simulink model "NonlinearNoObserverBlock"  (R2019b)
settings: Solver=VariableStepAuto  StartTime=0.0  StopTime=30  RelTol=1e-3
settings Model: Creator=marko  LastModifiedBy=marko

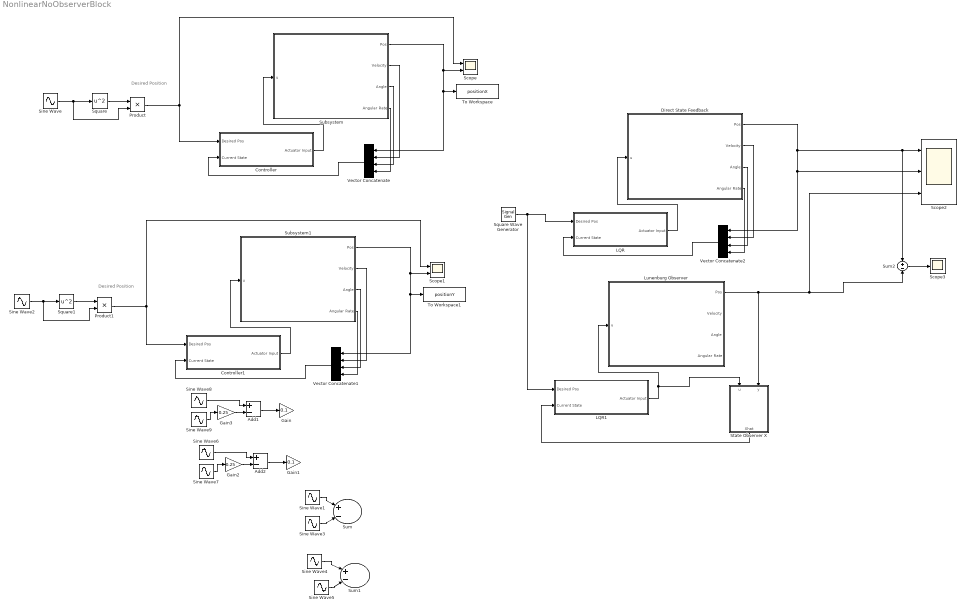
== system NonlinearNoObserverBlock ==
  note: Desired Position
  note: Desired Position
  Add1 : Sum  Inputs=+-
  Add2 : Sum  Inputs=+-
  Controller : Subsystem
  Controller1 : Subsystem
  Direct State Feedback : Subsystem
  Gain : Gain  Gain=0.1
  Gain1 : Gain  Gain=0.1
  Gain2 : Gain  Gain=0.25
  Gain3 : Gain  Gain=0.25
  LQR : Subsystem
  LQR1 : Subsystem
  Lunenburg Observer : Subsystem
  Product : Product
  Product1 : Product
  Scope : Scope  NumInputPorts=2
  Scope1 : Scope  NumInputPorts=2
  Scope2 : Scope  NumInputPorts=3
  Scope3 : Scope
  Sine Wave : Sin  SampleTime=0
  Sine Wave1 : Sin  Amplitude=2  SampleTime=0
  Sine Wave2 : Sin  Phase=pi/2  SampleTime=0
  Sine Wave3 : Sin  Frequency=2  SampleTime=0
  Sine Wave4 : Sin  Amplitude=2  Phase=pi/2  SampleTime=0
  Sine Wave5 : Sin  Frequency=2  Phase=pi/2  SampleTime=0
  Sine Wave6 : Sin  Amplitude=1.25  Phase=pi/2  SampleTime=0
  Sine Wave7 : Sin  Frequency=5  Phase=pi/2  SampleTime=0
  Sine Wave8 : Sin  Amplitude=1.25  Phase=pi/2  SampleTime=0
  Sine Wave9 : Sin  Frequency=5  Phase=pi/2  SampleTime=0
  Square : Math  Operator=square  SignedPower=off  SaturateOnIntegerOverflow=on
  Square Wave Generator : SignalGenerator  WaveForm=square  Amplitude=0.1  Frequency=0.5  Units=rad/sec
  Square1 : Math  Operator=square  SignedPower=off  SaturateOnIntegerOverflow=on
  State Observer X : Subsystem
  Subsystem : Subsystem
  Subsystem1 : Subsystem
  Sum : Sum  Inputs=|+-|
  Sum1 : Sum  Inputs=|+-|
  Sum2 : Sum  Inputs=+-
  To Workspace : ToWorkspace  VariableName=positionX  SampleTime=-1
  To Workspace1 : ToWorkspace  VariableName=positionY  SampleTime=-1
  Vector Concatenate : Concatenate  NumInputs=4
  Vector Concatenate1 : Concatenate  NumInputs=4
  Vector Concatenate2 : Concatenate  NumInputs=4
  wires:
  Subsystem/1(Pos) -> Scope/2, Vector Concatenate/1, To Workspace/1
  Controller/1(Actuator Input) -> Subsystem/1(u)
  Square1/1 -> Product1/1
  Product/1 -> Scope/1, Controller/1(Desired Pos)
  Sine Wave2/1 -> Product1/2, Square1/1
  Sine Wave4/1 -> Sum1/1
  Sine Wave3/1 -> Sum/2
  Sine Wave1/1 -> Sum/1
  Square/1 -> Product/1
  Sine Wave5/1 -> Sum1/2
  Sine Wave/1 -> Product/2, Square/1
  Vector Concatenate/1 -> Controller/2(Current State)
  Subsystem/2(Velocity) -> Vector Concatenate/2
  Subsystem/3(Angle) -> Vector Concatenate/3
  Subsystem/4(Angular Rate) -> Vector Concatenate/4
  Product1/1 -> Controller1/1(Desired Pos), Scope1/1
  Controller1/1(Actuator Input) -> Subsystem1/1(u)
  Vector Concatenate1/1 -> Controller1/2(Current State)
  Subsystem1/4(Angular Rate) -> Vector Concatenate1/4
  Subsystem1/1(Pos) -> Scope1/2, To Workspace1/1, Vector Concatenate1/1
  Subsystem1/3(Angle) -> Vector Concatenate1/3
  Subsystem1/2(Velocity) -> Vector Concatenate1/2
  Sine Wave7/1 -> Gain2/1
  Add2/1 -> Gain1/1
  Gain2/1 -> Add2/2
  Sine Wave6/1 -> Add2/1
  Gain3/1 -> Add1/2
  Sine Wave8/1 -> Add1/1
  Add1/1 -> Gain/1
  Sine Wave9/1 -> Gain3/1
  Direct State Feedback/3(Angle) -> Vector Concatenate2/3
  Direct State Feedback/2(Velocity) -> Vector Concatenate2/2
  LQR/1(Actuator Input) -> Direct State Feedback/1(u)
  Vector Concatenate2/1 -> LQR/2(Current State)
  Direct State Feedback/4(Angular Rate) -> Vector Concatenate2/4
  Direct State Feedback/1(Pos) -> Vector Concatenate2/1, Scope2/2, Sum2/1, Scope2/1
  LQR1/1(Actuator Input) -> State Observer X/1(u), Lunenburg Observer/1(u)
  State Observer X/1(Xhat) -> LQR1/2(Current State)
  Lunenburg Observer/1(Pos) -> State Observer X/2(y), Scope2/3, Sum2/2
  Sum2/1 -> Scope3/1
  Square Wave Generator/1 -> LQR1/1(Desired Pos), LQR/1(Desired Pos)

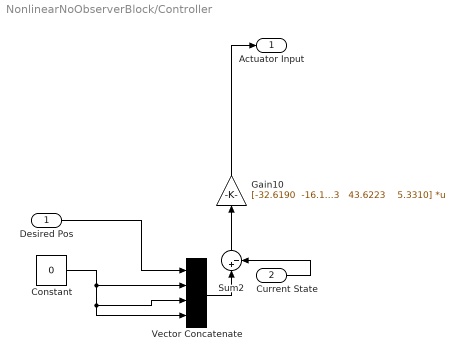
== system NonlinearNoObserverBlock/Controller ==
  Desired Pos : Inport
  Current State : Inport  Port=2
  Constant : Constant  Value=0
  Gain10 : Gain  Gain="[-32.6190  -16.1083   43.6223    5.3310]"  Multiplication=Matrix(K*u)
  Sum2 : Sum  Inputs=|+-
  Vector Concatenate : Concatenate  NumInputs=4
  Actuator Input : Outport
  wires:
  Desired Pos/1 -> Vector Concatenate/1
  Gain10/1 -> Actuator Input/1
  Constant/1 -> Vector Concatenate/2, Vector Concatenate/4, Vector Concatenate/3
  Current State/1 -> Sum2/2
  Sum2/1 -> Gain10/1
  Vector Concatenate/1 -> Sum2/1

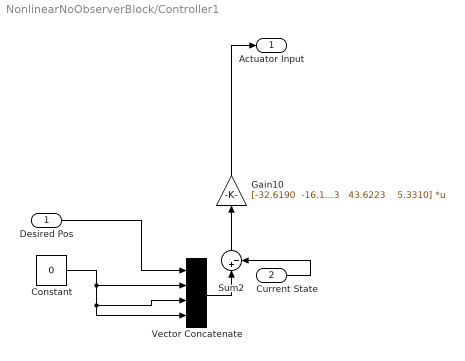
== system NonlinearNoObserverBlock/Controller1 ==
  Desired Pos : Inport
  Current State : Inport  Port=2
  Constant : Constant  Value=0
  Gain10 : Gain  Gain="[-32.6190  -16.1083   43.6223    5.3310]"  Multiplication=Matrix(K*u)
  Sum2 : Sum  Inputs=|+-
  Vector Concatenate : Concatenate  NumInputs=4
  Actuator Input : Outport
  wires:
  Desired Pos/1 -> Vector Concatenate/1
  Gain10/1 -> Actuator Input/1
  Constant/1 -> Vector Concatenate/2, Vector Concatenate/4, Vector Concatenate/3
  Current State/1 -> Sum2/2
  Sum2/1 -> Gain10/1
  Vector Concatenate/1 -> Sum2/1

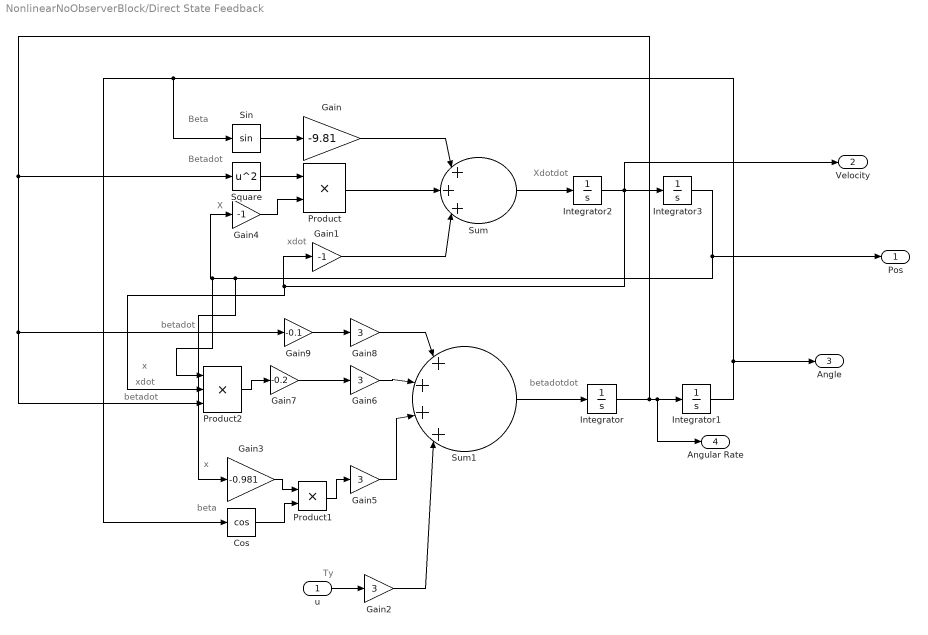
== system NonlinearNoObserverBlock/Direct State Feedback ==
  note: betadotdot
  note: betadot
  note: betadot
  note: xdot
  note: x
  note: beta
  note: x
  note: Ty
  note: xdot
  note: X
  note: Betadot
  note: Beta
  note: Xdotdot
  u : Inport
  Cos : Trigonometry  Operator=cos
  Gain : Gain  Gain=-9.81
  Gain1 : Gain  Gain=-1
  Gain{2,5..6,8} (4 alike) : Gain  Gain=3
  Gain3 : Gain  Gain=-0.981
  Gain4 : Gain  Gain=-1
  Gain7 : Gain  Gain=-0.2
  Gain9 : Gain  Gain=-0.1
  Integrator{,1..3} (4 alike) : Integrator
  Product : Product
  Product1 : Product
  Product2 : Product  Inputs=3
  Sin : Trigonometry
  Square : Math  Operator=square  SignedPower=off  SaturateOnIntegerOverflow=on
  Sum : Sum  Inputs=|+++|
  Sum1 : Sum  Inputs=|++++|
  Pos : Outport
  Velocity : Outport  Port=2
  Angle : Outport  Port=3
  Angular Rate : Outport  Port=4
  wires:
  Gain2/1 -> Sum1/4
  Gain8/1 -> Sum1/1
  Sum1/1 -> Integrator/1
  Integrator3/1 -> Pos/1, Gain3/1, Product2/1, Gain4/1
  Product1/1 -> Gain5/1
  Gain1/1 -> Sum/3
  Product/1 -> Sum/2
  Gain4/1 -> Product/2
  Sum/1 -> Integrator2/1
  Square/1 -> Product/1
  Gain3/1 -> Product1/1
  Gain6/1 -> Sum1/2
  Gain9/1 -> Gain8/1
  Gain/1 -> Sum/1
  Cos/1 -> Product1/2
  Integrator/1 -> Gain9/1, Product2/3, Square/1, Angular Rate/1, Integrator1/1
  Integrator1/1 -> Angle/1, Cos/1, Sin/1
  Gain5/1 -> Sum1/3
  Gain7/1 -> Gain6/1
  Sin/1 -> Gain/1
  Integrator2/1 -> Velocity/1, Product2/2, Gain1/1, Integrator3/1
  Product2/1 -> Gain7/1
  u/1 -> Gain2/1

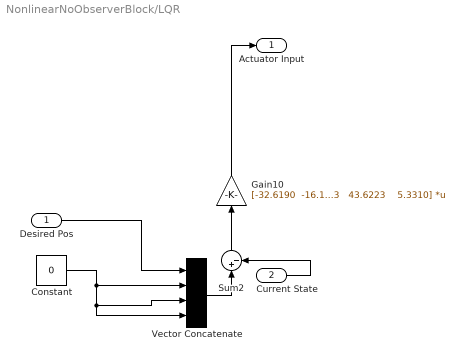
== system NonlinearNoObserverBlock/LQR ==
  Desired Pos : Inport
  Current State : Inport  Port=2
  Constant : Constant  Value=0
  Gain10 : Gain  Gain="[-32.6190  -16.1083   43.6223    5.3310]"  Multiplication=Matrix(K*u)
  Sum2 : Sum  Inputs=|+-
  Vector Concatenate : Concatenate  NumInputs=4
  Actuator Input : Outport
  wires:
  Desired Pos/1 -> Vector Concatenate/1
  Gain10/1 -> Actuator Input/1
  Constant/1 -> Vector Concatenate/2, Vector Concatenate/4, Vector Concatenate/3
  Current State/1 -> Sum2/2
  Sum2/1 -> Gain10/1
  Vector Concatenate/1 -> Sum2/1

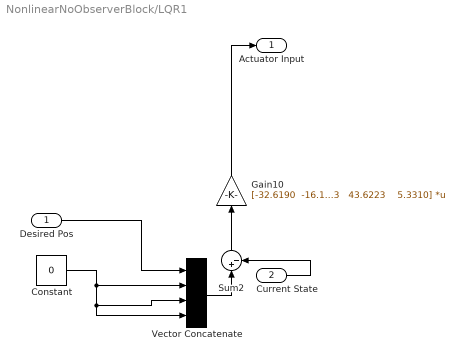
== system NonlinearNoObserverBlock/LQR1 ==
  Desired Pos : Inport
  Current State : Inport  Port=2
  Constant : Constant  Value=0
  Gain10 : Gain  Gain="[-32.6190  -16.1083   43.6223    5.3310]"  Multiplication=Matrix(K*u)
  Sum2 : Sum  Inputs=|+-
  Vector Concatenate : Concatenate  NumInputs=4
  Actuator Input : Outport
  wires:
  Desired Pos/1 -> Vector Concatenate/1
  Gain10/1 -> Actuator Input/1
  Constant/1 -> Vector Concatenate/2, Vector Concatenate/4, Vector Concatenate/3
  Current State/1 -> Sum2/2
  Sum2/1 -> Gain10/1
  Vector Concatenate/1 -> Sum2/1

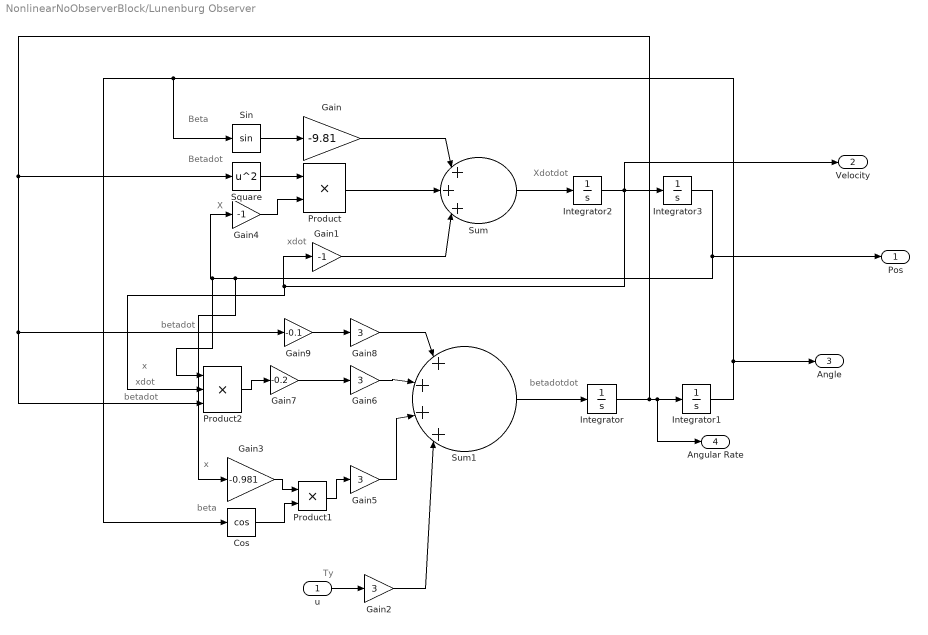
== system NonlinearNoObserverBlock/Lunenburg Observer ==
  note: betadotdot
  note: betadot
  note: betadot
  note: xdot
  note: x
  note: beta
  note: x
  note: Ty
  note: xdot
  note: X
  note: Betadot
  note: Beta
  note: Xdotdot
  u : Inport
  Cos : Trigonometry  Operator=cos
  Gain : Gain  Gain=-9.81
  Gain1 : Gain  Gain=-1
  Gain{2,5..6,8} (4 alike) : Gain  Gain=3
  Gain3 : Gain  Gain=-0.981
  Gain4 : Gain  Gain=-1
  Gain7 : Gain  Gain=-0.2
  Gain9 : Gain  Gain=-0.1
  Integrator{,1..3} (4 alike) : Integrator
  Product : Product
  Product1 : Product
  Product2 : Product  Inputs=3
  Sin : Trigonometry
  Square : Math  Operator=square  SignedPower=off  SaturateOnIntegerOverflow=on
  Sum : Sum  Inputs=|+++|
  Sum1 : Sum  Inputs=|++++|
  Pos : Outport
  Velocity : Outport  Port=2
  Angle : Outport  Port=3
  Angular Rate : Outport  Port=4
  wires:
  Gain2/1 -> Sum1/4
  Gain8/1 -> Sum1/1
  Sum1/1 -> Integrator/1
  Integrator3/1 -> Pos/1, Gain3/1, Product2/1, Gain4/1
  Product1/1 -> Gain5/1
  Gain1/1 -> Sum/3
  Product/1 -> Sum/2
  Gain4/1 -> Product/2
  Sum/1 -> Integrator2/1
  Square/1 -> Product/1
  Gain3/1 -> Product1/1
  Gain6/1 -> Sum1/2
  Gain9/1 -> Gain8/1
  Gain/1 -> Sum/1
  Cos/1 -> Product1/2
  Integrator/1 -> Gain9/1, Product2/3, Square/1, Angular Rate/1, Integrator1/1
  Integrator1/1 -> Angle/1, Cos/1, Sin/1
  Gain5/1 -> Sum1/3
  Gain7/1 -> Gain6/1
  Sin/1 -> Gain/1
  Integrator2/1 -> Velocity/1, Product2/2, Gain1/1, Integrator3/1
  Product2/1 -> Gain7/1
  u/1 -> Gain2/1

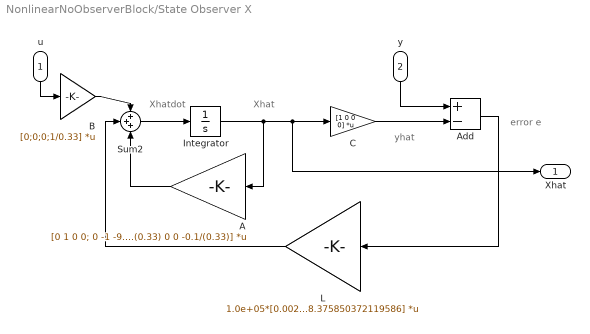
== system NonlinearNoObserverBlock/State Observer X ==
  note: Xhat
  note: error e
  note: yhat
  note: Xhatdot
  u : Inport
  y : Inport  Port=2
  A : Gain  Gain=[0 1 0 0; 0 -1 -9.8 0; 0 0 0 1; -0.98/(0.33) 0 0 -0.1/(0.33)]  Multiplication=Matrix(K*u)
  Add : Sum  Inputs=+-
  B : Gain  Gain=[0;0;0;1/0.33]  Multiplication=Matrix(K*u)
  C : Gain  Gain=[1 0 0 0]  Multiplication=Matrix(K*u)
  Integrator : Integrator  InitialCondition=[0;0;0;0]
  L : Gain  Gain=1.0e+05*[0.002186969696867;0.176147281894242; -0.645506052740811;-8.375850372119586]  Multiplication=Matrix(K*u)
  Sum2 : Sum  Inputs=+++
  Xhat : Outport
  wires:
  B/1 -> Sum2/1
  L/1 -> Sum2/2
  Integrator/1 -> A/1, C/1, Xhat/1
  Sum2/1 -> Integrator/1
  A/1 -> Sum2/3
  u/1 -> B/1
  C/1 -> Add/2
  y/1 -> Add/1
  Add/1 -> L/1

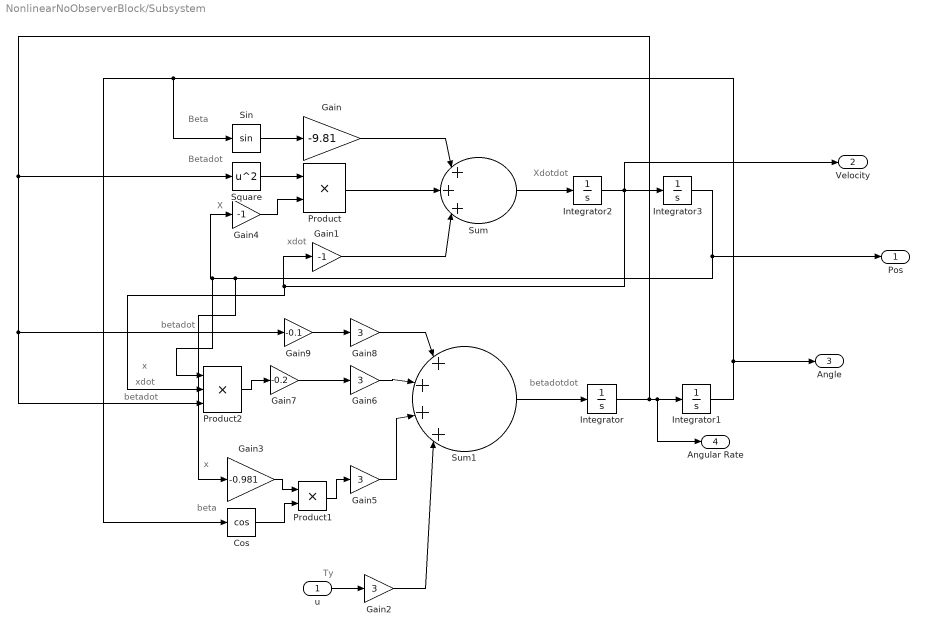
== system NonlinearNoObserverBlock/Subsystem ==
  note: betadotdot
  note: betadot
  note: betadot
  note: xdot
  note: x
  note: beta
  note: x
  note: Ty
  note: xdot
  note: X
  note: Betadot
  note: Beta
  note: Xdotdot
  u : Inport
  Cos : Trigonometry  Operator=cos
  Gain : Gain  Gain=-9.81
  Gain1 : Gain  Gain=-1
  Gain{2,5..6,8} (4 alike) : Gain  Gain=3
  Gain3 : Gain  Gain=-0.981
  Gain4 : Gain  Gain=-1
  Gain7 : Gain  Gain=-0.2
  Gain9 : Gain  Gain=-0.1
  Integrator{,1..3} (4 alike) : Integrator
  Product : Product
  Product1 : Product
  Product2 : Product  Inputs=3
  Sin : Trigonometry
  Square : Math  Operator=square  SignedPower=off  SaturateOnIntegerOverflow=on
  Sum : Sum  Inputs=|+++|
  Sum1 : Sum  Inputs=|++++|
  Pos : Outport
  Velocity : Outport  Port=2
  Angle : Outport  Port=3
  Angular Rate : Outport  Port=4
  wires:
  Gain2/1 -> Sum1/4
  Gain8/1 -> Sum1/1
  Sum1/1 -> Integrator/1
  Integrator3/1 -> Pos/1, Gain3/1, Product2/1, Gain4/1
  Product1/1 -> Gain5/1
  Gain1/1 -> Sum/3
  Product/1 -> Sum/2
  Gain4/1 -> Product/2
  Sum/1 -> Integrator2/1
  Square/1 -> Product/1
  Gain3/1 -> Product1/1
  Gain6/1 -> Sum1/2
  Gain9/1 -> Gain8/1
  Gain/1 -> Sum/1
  Cos/1 -> Product1/2
  Integrator/1 -> Gain9/1, Product2/3, Square/1, Angular Rate/1, Integrator1/1
  Integrator1/1 -> Angle/1, Cos/1, Sin/1
  Gain5/1 -> Sum1/3
  Gain7/1 -> Gain6/1
  Sin/1 -> Gain/1
  Integrator2/1 -> Velocity/1, Product2/2, Gain1/1, Integrator3/1
  Product2/1 -> Gain7/1
  u/1 -> Gain2/1

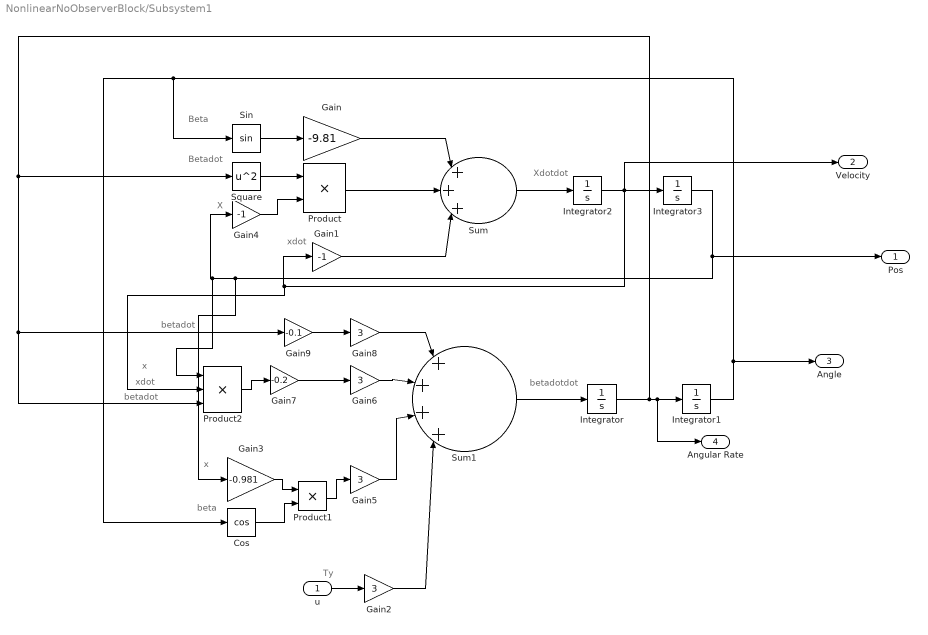
== system NonlinearNoObserverBlock/Subsystem1 ==
  note: betadotdot
  note: betadot
  note: betadot
  note: xdot
  note: x
  note: beta
  note: x
  note: Ty
  note: xdot
  note: X
  note: Betadot
  note: Beta
  note: Xdotdot
  u : Inport
  Cos : Trigonometry  Operator=cos
  Gain : Gain  Gain=-9.81
  Gain1 : Gain  Gain=-1
  Gain{2,5..6,8} (4 alike) : Gain  Gain=3
  Gain3 : Gain  Gain=-0.981
  Gain4 : Gain  Gain=-1
  Gain7 : Gain  Gain=-0.2
  Gain9 : Gain  Gain=-0.1
  Integrator{,1..3} (4 alike) : Integrator
  Product : Product
  Product1 : Product
  Product2 : Product  Inputs=3
  Sin : Trigonometry
  Square : Math  Operator=square  SignedPower=off  SaturateOnIntegerOverflow=on
  Sum : Sum  Inputs=|+++|
  Sum1 : Sum  Inputs=|++++|
  Pos : Outport
  Velocity : Outport  Port=2
  Angle : Outport  Port=3
  Angular Rate : Outport  Port=4
  wires:
  Gain2/1 -> Sum1/4
  Gain8/1 -> Sum1/1
  Sum1/1 -> Integrator/1
  Integrator3/1 -> Pos/1, Gain3/1, Product2/1, Gain4/1
  Product1/1 -> Gain5/1
  Gain1/1 -> Sum/3
  Product/1 -> Sum/2
  Gain4/1 -> Product/2
  Sum/1 -> Integrator2/1
  Square/1 -> Product/1
  Gain3/1 -> Product1/1
  Gain6/1 -> Sum1/2
  Gain9/1 -> Gain8/1
  Gain/1 -> Sum/1
  Cos/1 -> Product1/2
  Integrator/1 -> Gain9/1, Product2/3, Square/1, Angular Rate/1, Integrator1/1
  Integrator1/1 -> Angle/1, Cos/1, Sin/1
  Gain5/1 -> Sum1/3
  Gain7/1 -> Gain6/1
  Sin/1 -> Gain/1
  Integrator2/1 -> Velocity/1, Product2/2, Gain1/1, Integrator3/1
  Product2/1 -> Gain7/1
  u/1 -> Gain2/1
